simulink model "special_traj"  (R2018b)
settings: Solver=FixedStepDiscrete  StartTime=0.0  StopTime=10  FixedStep=Ts  RelTol=1e-3
InitFcn:
  | Ts = 0.001;
undefined symbols (not defined in the file or in its folder): DiscIntNeverNeededParam
libraries: powerlib_meascontrol x5, peGeneralControl x4
settings Model: Creator=Kamran  LastModifiedBy=Kamran
settings DebuggingCC: LibraryContextMissingDiagnostic=none
settings SFSimCC: SimUseLocalCustomCode=off
settings RTWCC: RTWUseLocalCustomCode=off

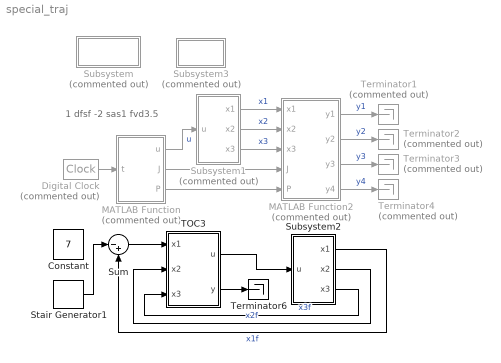
== system special_traj ==
  note: 1 dfsf -2 sas1 fvd3.5
  Constant : Constant  Value=7  SampleTime=Ts
  Digital Clock : DigitalClock  Commented=on  SampleTime=Ts
  MATLAB Function : MATLAB Function  Commented=on  TreatAsAtomicUnit=on
  MATLAB Function2 : MATLAB Function  Commented=on  TreatAsAtomicUnit=on
  Stair Generator1 : powerlib_meascontrol/Pulse & Signal Generators/Stair Generator  t=[0, 1, 5]  e=[1, 5, -3]  Ts=Ts
      settings: SourceProductName=Simscape Power Systems
  Subsystem : Subsystem  Commented=on
  Subsystem1 : Subsystem  Commented=on
  Subsystem2 : Subsystem  mask{X10=0, X20=0, X2M=inf, X30=0, X3M=1.5}
  Subsystem3 : Subsystem  Commented=on
  Sum : Sum  Inputs=|-+
  TOC3 : MATLAB Function  TreatAsAtomicUnit=on  SystemSampleTime=Ts
  Terminator{1..4} (4 alike) : Terminator  Commented=on
  Terminator6 : Terminator
  wires:
  MATLAB Function/1(u) -> Subsystem1/1(u)  "u"
  Digital Clock/1 -> MATLAB Function/1(t)
  MATLAB Function2/1(y1) -> Terminator1/1  "y1"
  Subsystem1/1(x1) -> MATLAB Function2/1(x1)  "x1"
  Subsystem1/2(x2) -> MATLAB Function2/2(x2)  "x2"
  Subsystem1/3(x3) -> MATLAB Function2/3(x3)  "x3"
  MATLAB Function2/2(y2) -> Terminator2/1  "y2"
  MATLAB Function/2(J) -> MATLAB Function2/4(J)
  MATLAB Function2/3(y3) -> Terminator3/1  "y3"
  MATLAB Function2/4(y4) -> Terminator4/1  "y4"
  MATLAB Function/3(P) -> MATLAB Function2/5(P)
  TOC3/1(u) -> Subsystem2/1(u)
  Subsystem2/1(x1) -> Sum/2  "x1f"
  Subsystem2/2(x2) -> TOC3/2(x2)  "x2f"
  Subsystem2/3(x3) -> TOC3/3(x3)  "x3f"
  TOC3/2(y) -> Terminator6/1
  Stair Generator1/1 -> Sum/1
  Sum/1 -> TOC3/1(x1)

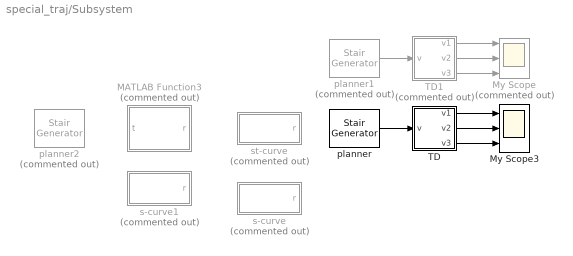
== system special_traj/Subsystem ==
  MATLAB Function3 : MATLAB Function  Commented=on  TreatAsAtomicUnit=on
  My Scope : Scope  Commented=on  NumInputPorts=3
  My Scope3 : Scope  NumInputPorts=3
  TD : Subsystem  mask{x3m=4, x2m=3}
      mask prompts: x3m "x3 max"; x2m "x2 max"
  TD1 : Subsystem  Commented=on  mask{J=1, A=1, D=0.5}
  planner : powerlib_meascontrol/Pulse & Signal Generators/Stair Generator  t=[0, 1, 4]  e=[0, 1, 0]  Ts=Ts
      settings: SourceProductName=Simscape Electrical
  planner1 : powerlib_meascontrol/Pulse & Signal Generators/Stair Generator  Commented=on  t=[0, 1, 5, 8]  e=[0, 1, 0.1, 0]  Ts=Ts
      settings: SourceProductName=Simscape Electrical
  planner2 : powerlib_meascontrol/Pulse & Signal Generators/Stair Generator  Commented=on  t=[0, 1.9, 6, 8.1]  e=[1, -1, 1, 0]  Ts=Ts
      settings: SourceProductName=Simscape Electrical
  s-curve : MATLAB Function  Commented=on  TreatAsAtomicUnit=on  mask{P=3, V=1, A=2, J=3, Ts=0.001}
  s-curve1 : MATLAB Function  Commented=on  TreatAsAtomicUnit=on  mask{P=0.5, V=1, A=1, D=2, J=3, I=6, Ts=0.001}
  st-curve : MATLAB Function  Commented=on  TreatAsAtomicUnit=on  mask{P=3, V=1, A=2, J=3, Ts=Ts}
  wires:
  TD/3(v3) -> My Scope3/3
  TD/2(v2) -> My Scope3/2
  TD1/2(v2) -> My Scope/2
  TD/1(v1) -> My Scope3/1
  planner1/1 -> TD1/1(v)
  TD1/3(v3) -> My Scope/3
  TD1/1(v1) -> My Scope/1
  planner/1 -> TD/1(v)

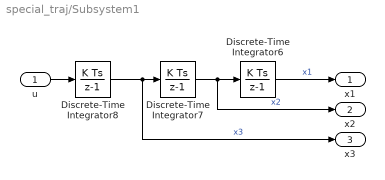
== system special_traj/Subsystem1 ==
  u : Inport
  Discrete-Time Integrator6 : DiscreteIntegrator  SampleTime=-1  ICPrevOutput=DiscIntNeverNeededParam  ICPrevScaledInput=DiscIntNeverNeededParam
  Discrete-Time Integrator7 : DiscreteIntegrator  SampleTime=-1  ICPrevOutput=DiscIntNeverNeededParam  ICPrevScaledInput=DiscIntNeverNeededParam
  Discrete-Time Integrator8 : DiscreteIntegrator  SampleTime=-1  ICPrevOutput=DiscIntNeverNeededParam  ICPrevScaledInput=DiscIntNeverNeededParam
  x1 : Outport
  x2 : Outport  Port=2
  x3 : Outport  Port=3
  wires:
  Discrete-Time Integrator8/1 -> x3/1, Discrete-Time Integrator7/1  "x3"
  Discrete-Time Integrator7/1 -> x2/1, Discrete-Time Integrator6/1  "x2"
  u/1 -> Discrete-Time Integrator8/1
  Discrete-Time Integrator6/1 -> x1/1  "x1"

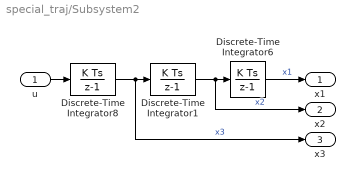
== system special_traj/Subsystem2 ==
  u : Inport
  Discrete-Time Integrator1 : DiscreteIntegrator  InitialCondition=X20  SampleTime=-1  LimitOutput=on  UpperSaturationLimit=X2M  LowerSaturationLimit=-X2M  ICPrevOutput=DiscIntNeverNeededParam  ICPrevScaledInput=DiscIntNeverNeededParam
  Discrete-Time Integrator6 : DiscreteIntegrator  InitialCondition=X10  SampleTime=-1  ICPrevOutput=DiscIntNeverNeededParam  ICPrevScaledInput=DiscIntNeverNeededParam
  Discrete-Time Integrator8 : DiscreteIntegrator  InitialCondition=X30  SampleTime=-1  LimitOutput=on  UpperSaturationLimit=X3M  LowerSaturationLimit=-X3M  ICPrevOutput=DiscIntNeverNeededParam  ICPrevScaledInput=DiscIntNeverNeededParam
  x1 : Outport
  x2 : Outport  Port=2
  x3 : Outport  Port=3
  wires:
  Discrete-Time Integrator8/1 -> x3/1, Discrete-Time Integrator1/1  "x3"
  Discrete-Time Integrator1/1 -> x2/1, Discrete-Time Integrator6/1  "x2"
  u/1 -> Discrete-Time Integrator8/1
  Discrete-Time Integrator6/1 -> x1/1  "x1"

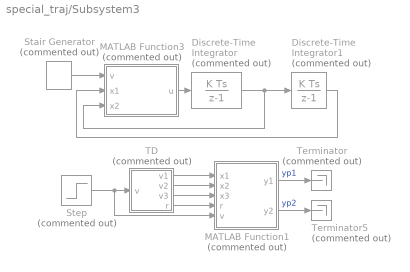
== system special_traj/Subsystem3 ==
  Discrete-Time Integrator : DiscreteIntegrator  Commented=on  SampleTime=-1  LimitOutput=on  UpperSaturationLimit=2  LowerSaturationLimit=-2  ICPrevOutput=DiscIntNeverNeededParam  ICPrevScaledInput=DiscIntNeverNeededParam
  Discrete-Time Integrator1 : DiscreteIntegrator  Commented=on  SampleTime=-1  ICPrevOutput=DiscIntNeverNeededParam  ICPrevScaledInput=DiscIntNeverNeededParam
  MATLAB Function1 : MATLAB Function  Commented=on  TreatAsAtomicUnit=on
  MATLAB Function3 : MATLAB Function  Commented=on  TreatAsAtomicUnit=on
  Stair Generator : powerlib_meascontrol/Pulse & Signal Generators/Stair Generator  Commented=on  t=[0, 1, 4]  e=[1, 5, -3]  Ts=Ts
      settings: SourceProductName=Simscape Power Systems
  Step : Step  Commented=on  After=3  SampleTime=Ts
  TD : Subsystem  Commented=on  mask{x3m=2, x2m=inf}
      mask prompts: x3m "x3 max"; x2m "x2 max"
  Terminator : Terminator  Commented=on
  Terminator5 : Terminator  Commented=on
  wires:
  Discrete-Time Integrator/1 -> MATLAB Function3/3(x2), Discrete-Time Integrator1/1
  Discrete-Time Integrator1/1 -> MATLAB Function3/2(x1)
  MATLAB Function3/1(u) -> Discrete-Time Integrator/1
  Stair Generator/1 -> MATLAB Function3/1(v)
  TD/4(r) -> MATLAB Function1/4(r)
  Step/1 -> MATLAB Function1/5(v), TD/1(v)
  TD/1(v1) -> MATLAB Function1/1(x1)
  MATLAB Function1/2(y2) -> Terminator5/1  "yp2"
  MATLAB Function1/1(y1) -> Terminator/1  "yp1"
  TD/2(v2) -> MATLAB Function1/2(x2)
  TD/3(v3) -> MATLAB Function1/3(x3)

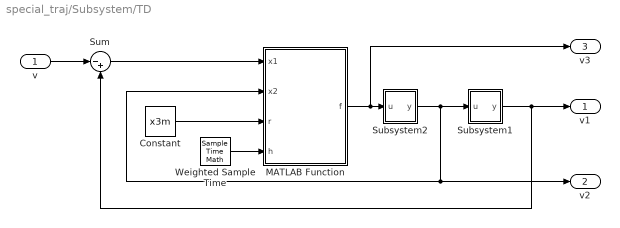
== system special_traj/Subsystem/TD ==
  v : Inport
  Constant : Constant  Value=x3m  SampleTime=-1
  MATLAB Function : MATLAB Function  TreatAsAtomicUnit=on
  Subsystem1 : Subsystem  mask{sat=inf, x0=0}
      mask Display: droots([], [0], 1);
  Subsystem2 : Subsystem  mask{sat=x2m, x0=0}
      mask Display: droots([], [0], 1);
  Sum : Sum  Inputs=|-+
  Weighted Sample Time : SampleTimeMath  TsampMathOp=Ts Only
  v1 : Outport
  v2 : Outport  Port=2
  v3 : Outport  Port=3
  wires:
  Subsystem2/1(y) -> Subsystem1/1(u), v2/1, MATLAB Function/2(x2)
  Subsystem1/1(y) -> Sum/2, v1/1
  v/1 -> Sum/1
  Weighted Sample Time/1 -> MATLAB Function/4(h)
  Sum/1 -> MATLAB Function/1(x1)
  Constant/1 -> MATLAB Function/3(r)
  MATLAB Function/1(f) -> v3/1, Subsystem2/1(u)

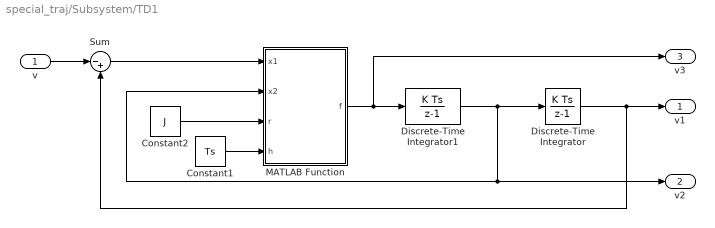
== system special_traj/Subsystem/TD1 ==
  v : Inport
  Constant1 : Constant  Value=Ts  SampleTime=-1
  Constant2 : Constant  Value=J  SampleTime=-1
  Discrete-Time Integrator : DiscreteIntegrator  SampleTime=-1  ICPrevOutput=DiscIntNeverNeededParam  ICPrevScaledInput=DiscIntNeverNeededParam
  Discrete-Time Integrator1 : DiscreteIntegrator  SampleTime=-1  LimitOutput=on  UpperSaturationLimit=A  LowerSaturationLimit=-D  ICPrevOutput=DiscIntNeverNeededParam  ICPrevScaledInput=DiscIntNeverNeededParam
  MATLAB Function : MATLAB Function  TreatAsAtomicUnit=on
  Sum : Sum  Inputs=|-+
  v1 : Outport
  v2 : Outport  Port=2
  v3 : Outport  Port=3
  wires:
  Discrete-Time Integrator/1 -> Sum/2, v1/1
  v/1 -> Sum/1
  Constant1/1 -> MATLAB Function/4(h)
  Sum/1 -> MATLAB Function/1(x1)
  MATLAB Function/1(f) -> v3/1, Discrete-Time Integrator1/1
  Discrete-Time Integrator1/1 -> Discrete-Time Integrator/1, v2/1, MATLAB Function/2(x2)
  Constant2/1 -> MATLAB Function/3(r)

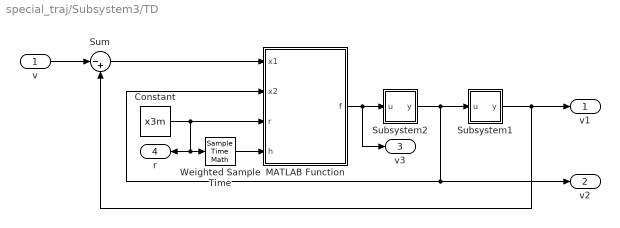
== system special_traj/Subsystem3/TD ==
  v : Inport
  Constant : Constant  Value=x3m  SampleTime=-1
  MATLAB Function : MATLAB Function  TreatAsAtomicUnit=on
  Subsystem1 : Subsystem  mask{sat=inf, x0=0}
      mask Display: droots([], [0], 1);
  Subsystem2 : Subsystem  mask{sat=x2m, x0=0}
      mask Display: droots([], [0], 1);
  Sum : Sum  Inputs=|-+
  Weighted Sample Time : SampleTimeMath  TsampMathOp=Ts Only
  v1 : Outport
  v2 : Outport  Port=2
  v3 : Outport  Port=3
  r : Outport  Port=4
  wires:
  Subsystem2/1(y) -> Subsystem1/1(u), v2/1, MATLAB Function/2(x2)
  Subsystem1/1(y) -> Sum/2, v1/1
  v/1 -> Sum/1
  Weighted Sample Time/1 -> MATLAB Function/4(h)
  Sum/1 -> MATLAB Function/1(x1)
  MATLAB Function/1(f) -> v3/1, Subsystem2/1(u)
  Constant/1 -> r/1, Weighted Sample Time/1, MATLAB Function/3(r)

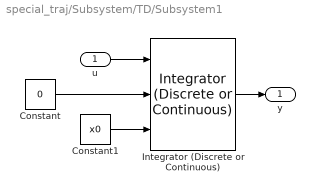
== system special_traj/Subsystem/TD/Subsystem1 ==
  u : Inport
  Constant : Constant  Value=0
  Constant1 : Constant  Value=x0
  Integrator (Discrete or Continuous) : peGeneralControl/Integrator (Discrete or Continuous)  LabelModeActiveChoice=Discrete  ExternalReset=level  LimitType=Anti-windup  B=sat  A=-sat  Ts=-1
  y : Outport
  wires:
  Constant1/1 -> Integrator (Discrete or Continuous)/3
  u/1 -> Integrator (Discrete or Continuous)/1
  Constant/1 -> Integrator (Discrete or Continuous)/2
  Integrator (Discrete or Continuous)/1 -> y/1

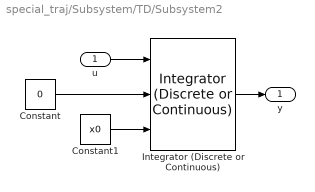
== system special_traj/Subsystem/TD/Subsystem2 ==
  u : Inport
  Constant : Constant  Value=0
  Constant1 : Constant  Value=x0
  Integrator (Discrete or Continuous) : peGeneralControl/Integrator (Discrete or Continuous)  LabelModeActiveChoice=Discrete  ExternalReset=level  LimitType=Anti-windup  B=sat  A=-sat  Ts=-1
  y : Outport
  wires:
  Integrator (Discrete or Continuous)/1 -> y/1
  Constant/1 -> Integrator (Discrete or Continuous)/2
  u/1 -> Integrator (Discrete or Continuous)/1
  Constant1/1 -> Integrator (Discrete or Continuous)/3

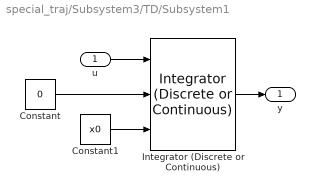
== system special_traj/Subsystem3/TD/Subsystem1 ==
  u : Inport
  Constant : Constant  Value=0
  Constant1 : Constant  Value=x0
  Integrator (Discrete or Continuous) : peGeneralControl/Integrator (Discrete or Continuous)  LabelModeActiveChoice=Discrete  ExternalReset=level  LimitType=Anti-windup  B=sat  A=-sat  Ts=-1
  y : Outport
  wires:
  Constant1/1 -> Integrator (Discrete or Continuous)/3
  u/1 -> Integrator (Discrete or Continuous)/1
  Constant/1 -> Integrator (Discrete or Continuous)/2
  Integrator (Discrete or Continuous)/1 -> y/1

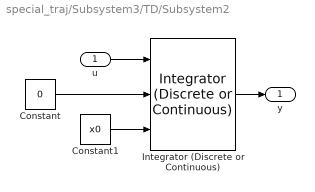
== system special_traj/Subsystem3/TD/Subsystem2 ==
  u : Inport
  Constant : Constant  Value=0
  Constant1 : Constant  Value=x0
  Integrator (Discrete or Continuous) : peGeneralControl/Integrator (Discrete or Continuous)  LabelModeActiveChoice=Discrete  ExternalReset=level  LimitType=Anti-windup  B=sat  A=-sat  Ts=-1
  y : Outport
  wires:
  Integrator (Discrete or Continuous)/1 -> y/1
  Constant/1 -> Integrator (Discrete or Continuous)/2
  u/1 -> Integrator (Discrete or Continuous)/1
  Constant1/1 -> Integrator (Discrete or Continuous)/3

== matlab function special_traj/Subsystem/s-curve1 ==
  data: r output; P parameter; V parameter; A parameter; D parameter; J parameter; I parameter; Ts parameter
function r = profile(P, V, A, D, J, I, Ts)

persistent t;
if isempty(t)
    t = 0;
else
    t = t + Ts;
end

if P/V < (A/J/2 + V/A/2 + D/I/2 + V/D/2)
    a = 1/A + 1/D;
    b = A/J + D/I;
    c = -2*P;
    V = -b + sqrt(b^2 - 4*a*c)/2/a;
end

if V*J < A^2
    A = sqrt(V*J);
end

if V*I < D^2
    D = sqrt(V*I);
end

t1 = A/J;
t2 = V/A - A/J;
t3 = P/V - A/J/2 - V/A/2 - D/I/2 - V/D/2;
t4 = D/I;
t5 = V/D - D/I;

% t1 = A/J;
% t4 = D/I;
% t2 = V/A - t1;
% t5 = V/D - t4;
% t3 = P/V - t2/2 - t1 - t5/2 - t4;

% t  = round(t  / Ts) * Ts;
t1 = round(t1 / Ts) * Ts;
t2 = round(t2 / Ts) * Ts;
t3 = round(t3 / Ts) * Ts;
t4 = round(t4 / Ts) * Ts;
t5 = round(t5 / Ts) * Ts;

% K = 2*P/(t1*(t1+t2)*(t5+2*t4+2*t3+2*t1+t2));

if 0
elseif t < (t1)
    r = +J;
elseif t < (t1 + t2)
    r = 0;
elseif t < (2*t1 + t2)
    r = -J;
elseif t < (2*t1 + t2 + t3)
    r = 0;
elseif t < (2*t1 + t2 + t3 + t4)
    r = -I;
elseif t < (2*t1 + t2 + t3 + t4 + t5)
    r = 0;
elseif t < (2*t1 + t2 + t3 + 2*t4 + t5)
    r = I;
else
    r = 0;
end

end

== matlab function special_traj/Subsystem/TD1/MATLAB Function ==
  data: x1 input; f output; x2 input; r input; h input
function f = fhan(x1, x2, r, h)

    d = r * h^2;
    a0 = h * x2;
    y = x1 + a0;
    a1 = sqrt(d * (d + 8 * abs(y)));
    a2 = a0 + sign(y) * (a1 - d) / 2;
    sy = (sign(y + d) - sign(y - d)) / 2;
    a = (a0 + y - a2) * sy + a2;
    sa = (sign(a + d) - sign(a - d)) / 2;
    f = -r * (a / d - sign(a)) * sa - r * sign(a);

end

== matlab function special_traj/Subsystem/s-curve ==
  data: r output; P parameter; V parameter; A parameter; J parameter; Ts parameter
function r = profile(P, V, A, J, Ts)

persistent t;
if isempty(t)
    t = 0;
else
    t = t + Ts;
end

if P/V < (A/J + V/A)
    b = A/J;
    V = A * (-b + sqrt(b^2 + 4*P/A)) / 2;
end

if V*J < A^2
    A = sqrt(J*V);
end

t1 = A/J;
t2 = V/A - A/J;
t3 = P/V - V/A - A/J;
t4 = t1;
t5 = t2;

t = round(t / Ts) * Ts;
t1 = round(t1 / Ts) * Ts;
t2 = round(t2 / Ts) * Ts;
t3 = round(t3 / Ts) * Ts;
t4 = round(t4 / Ts) * Ts;
t5 = round(t5 / Ts) * Ts;

K = 2*P/(t1*(t1+t2)*(t5+2*t4+2*t3+2*t1+t2));

if 0
elseif t < (t1)
    r = +K;
elseif t < (t1 + t2)
    r = 0;
elseif t < (2*t1 + t2)
    r = -K;
elseif t < (2*t1 + t2 + t3)
    r = 0;
elseif t < (2*t1 + t2 + t3 + t4)
    r = -K;
elseif t < (2*t1 + t2 + t3 + t4 + t5)
    r = 0;
elseif t < (2*t1 + t2 + t3 + 2*t4 + t5)
    r = K;
else
    r = 0;
end

end

== matlab function special_traj/Subsystem/TD/MATLAB Function ==
  data: x1 input; f output; x2 input; r input; h input
function f = fhan(x1, x2, r, h)

    d = r * h^2;
    a0 = h * x2;
    y = x1 + a0;
    a1 = sqrt(d * (d + 8 * abs(y)));
    a2 = a0 + sign(y) * (a1 - d) / 2;
    sy = (sign(y + d) - sign(y - d)) / 2;
    a = (a0 + y - a2) * sy + a2;
    sa = (sign(a + d) - sign(a - d)) / 2;
    f = -r * (a / d - sign(a)) * sa - r * sign(a);

end

== matlab function special_traj/Subsystem/MATLAB Function3 ==
  data: t input; r output
function r = fcn(t)

P = 15;
J = 1;
I = J;
A = 1;
D = A;
V = 1;

t1 = A/J;
t2 = V/A - A/J;
t3 = P/V - A/J/2 - V/A/2 - D/I/2 - V/D/2;
t4 = D/I;
t5 = V/D - D/I;

ro = D/A;
con1 = V >= (A^2/J);
con2 = V >= (D^2/I);
con3 = P/V >= (D/2/J/ro + ro*V/2/D + D/2/J + V/2/D);
con4 = P/V >= ((1+1/ro)*D/2/J + (ro+1)*V/2/D);

if ~con1 || ~con2 || ~con3 || ~con4
    r = 0;
elseif t < (t1)
    r = +1;
elseif t < (t1 + t2)
    r = 0;
elseif t < (2*t1 + t2)
    r = -1;
elseif t < (2*t1 + t2 + t3)
    r = 0;
elseif t < (2*t1 + t2 + t3 + t4)
    r = -1;
elseif t < (2*t1 + t2 + t3 + t4 + t5)
    r = 0;
elseif t < (2*t1 + t2 + t3 + 2*t4 + t5)
    r = 1;
else
    r = 0;
end

end

== matlab function special_traj/Subsystem/st-curve ==
  data: r output; P parameter; V parameter; A parameter; J parameter; Ts parameter
function r = profile(P, V, A, J, Ts)

persistent t;
if isempty(t)
    t = 0;
else
    t = t + Ts;
end

if P/V < 3*A/2/J + V/A
    b = 3*A/2/J;
    V = A * (-b + sqrt(b^2 + 4*P/A)) / 2;
end

if 2*J*V < 3*A^2
    A = sqrt(2*J*V/3);
end

t1 = 3*A/2/J;
t2 = V/A - t1;
t3 = P/V - V/A - t1;
t4 = t1;
t5 = t2;

t = round(t / Ts) * Ts;
t1 = round(t1 / Ts) * Ts;
t2 = round(t2 / Ts) * Ts;
t3 = round(t3 / Ts) * Ts;
t4 = round(t4 / Ts) * Ts;
t5 = round(t5 / Ts) * Ts;

K = 12*P/(t1^3*(t1+t2)*(t5+2*t4+2*t3+2*t1+t2));

if 0
elseif t < (t1)
    tt = t;
    ss = tt*(t1-tt);
    r = +K*ss;
elseif t < (t1 + t2)
    r = 0;
elseif t < (2*t1 + t2)
    tt = t - (t1 + t2);
    ss = tt*(t1-tt);
    r = -K*ss;
elseif t < (2*t1 + t2 + t3)
    r = 0;
elseif t < (2*t1 + t2 + t3 + t4)
    tt = t - (2*t1 + t2 + t3);
    ss = tt*(t1-tt);
    r = -K*ss;
elseif t < (2*t1 + t2 + t3 + t4 + t5)
    r = 0;
elseif t < (2*t1 + t2 + t3 + 2*t4 + t5)
    tt = t - (2*t1 + t2 + t3 + t4 + t5);
    ss = tt*(t1-tt);
    r = K*ss;
else
    r = 0;
end

end

== matlab function special_traj/MATLAB Function ==
  data: t input; u output; J output; P output
function [u, J, P] = fcn(t)

S = 1;
P = 6*S;
J = 4*S;
O = 0;
T = nthroot(P/J/2,3);

t = t - O;

if (t<0)
    u = 0;
elseif (t<T)
    u = +J;
elseif (t<3*T)
    u = -J;
elseif (t<4*T)
    u = +J;
else
    u = 0;
end

== matlab function special_traj/Subsystem3/TD/MATLAB Function ==
  data: x1 input; f output; x2 input; r input; h input
function f = fhan(x1, x2, r, h)

    d = r * h^2;
    a0 = h * x2;
    y = x1 + a0;
    a1 = sqrt(d * (d + 8 * abs(y)));
    a2 = a0 + sign(y) * (a1 - d) / 2;
    sy = (sign(y + d) - sign(y - d)) / 2;
    a = (a0 + y - a2) * sy + a2;
    sa = (sign(a + d) - sign(a - d)) / 2;
    f = -r * (a / d - sign(a)) * sa - r * sign(a);
    
%     f = -sign(x1 + .5*x2*abs(x2));

end

== matlab function special_traj/Subsystem3/MATLAB Function1 ==
  data: x1 input; x2 input; x3 input; r input; y1 output; v input; y2 output
function [y1, y2] = fcn(x1, x2, x3, r, v)
%   y = -sat(x1 - v + x2*abs(x2)/2);
    e = v - x1;
    
    y1 = -e + x2*abs(x2)/2/r;
    y2 = -e - x2*abs(x2)/2/r;
    
%     y1 = -e + x2^2/2;
%     y2 = -e - x2^2/2;
end

function y = sat(s)
    psi = eps;
    if (abs(s) > psi)
        y = sign(s);
    else
        y = s / psi;
    end
end

== matlab function special_traj/MATLAB Function2 ==
  data: x1 input; x2 input; x3 input; J input; y1 output; y2 output; y3 output; y4 output; P input
function [y1, y2, y3, y4] = fcn(x1, x2, x3, J, P)
    r = abs(J);
    e = P - x1;
    
    y1 = -e + x3^3/3/r^2 + x3*abs(x2)/r;
    y2 = -e + x3^3/3/r^2 - x3*abs(x2)/r;
    
    y3 = x2 + x3*abs(x3)/2/r;
    y4 = x2 - x3*abs(x3)/2/r;
    
    y3 = sign(x2) * (abs(x2) + x3^2/2/r);
    y4 = sign(x2) * (abs(x2) - x3^2/2/r);
    
    xc = y1 + y3*sqrt(abs(y3)/r);
    
%     y1 = -e + x3^3/3/r^2 + x2*x3/r;
%     y2 = -e + x3^3/3/r^2 - x2*x3/r;
%     y3 = x2 + x3^2/2/r;
%     y4 = x2 - x3^2/2/r;
end

== matlab function special_traj/TOC3 ==
  data: u output; x1 input; x2 input; x3 input; y output
function [u, y] = fcn(x1, x2, x3)
    r = 2.5;
    h = 0.001;
    vm = 2.5;
    
    y1 = x1  + x3^3/3/r^2 + x3*abs(x2)/r;
    y3 = sign(x2) * (abs(x2) + x3^2/2/r);
    pcan = y3*sqrt(abs(y3)/r);
    xcal = y1 + pcan;
    y4 = x2 + x3*abs(x3)/2/r;
    y = [xcal y4];
    
%     u = fhan(x2, x3, r, h);
    
    if abs(y3) > vm && sign(x2) == sign(x3)
        u = -r*sign(y3);
    elseif abs(xcal) > 0.5
        u = -r * sign(xcal);
    else
        u = fhan(x2, x3, r, h);
%         u = -r * sign(y4);
    end

%     b1 = xcalc(-e+x2*h*2, x2+x3*h*2, x3+r*h*2, 0.9*r);% estimate(-e, x2, x3, -r, r*1.1, h);
%     b2 = xcalc(-e+x2*h*2, x2+x3*h*2, x3+r*h*2, 1.1*r);% estimate(-e, x2, x3, -r, r*0.9, h);
%     kk=r;
%    if(sign(b1)~=sign(b2))
%         kk =  (1-0.1*(b1 + b2) / (b1 - b2))*r;
%    end
%    
%     a1 = estimate(-e, x2, x3, +kk, kk, h);
%     a2 = estimate(-e, x2, x3, -kk, kk, h);
%     a0 = estimate(-e, x2, x3,  0, kk, h);
% 
%     y = [a1 a2 a0 b1 b2 kk];
% 
%         u = -kk * (a1 + a2) / (a1 - a2);
%         if abs(u) > kk
%             u = kk * sign(u);
%         end

    %if(sign(a1)==sign(a2))
    %    u= -r*sign(abs(a1)-abs(a2))*1.02;
    %else
            %u=-(abs(a1)*r+abs(a2)*-r)/(abs(a1)+abs(a2));
    %end
    
%     if abs(y3) > vm && sign(y3) == sign(x3)
%         u = -r*sign(y3);
%     elseif abs(xcal) > 0.05
%         u = -r * sign(xcal);
%     else
%         u = fhan(x2, x3, r, h);
% %         u = -r * sign(y4);
%     end
end

function xc = estimate1(x1, x2, x3, rs, jmax, h)
    d1 = x1 + x2 * h;
    d2 = x2 + x3 * h;
    d3 = x3 + rs * h;
    xc = xcalc(d1, d2, d3, jmax);
end

function xc = estimate2(x1, x2, x3, rs, jmax, h)
    d1 = x1 + x2 * h;
    d2 = x2 + x3 * h;
    d3 = x3 + rs * h;
    d1 = d1 + d2 * h;
    d2 = d2 + d3 * h;
    d3 = d3 - rs * h;
    xc = xcalc(d1, d2, d3, jmax);
end

function xc = xcalc(x1, x2, x3, r)
    y1 = x1 + x3^3/3/r^2 + x3*abs(x2)/r;
    y3 = sign(x2) * (abs(x2) + x3^2/2/r);
    xc = y1 + y3*sqrt(abs(y3)/r);
end

function f = fhan(x1, x2, r, h)
    d = r * h^2;
    a0 = h * x2;
    y = x1 + a0;
    a1 = sqrt(d * (d + 8 * abs(y)));
    a2 = a0 + sign(y) * (a1 - d) / 2;
    sy = (sign(y + d) - sign(y - d)) / 2;
    a = (a0 + y - a2) * sy + a2;
    sa = (sign(a + d) - sign(a - d)) / 2;
    f = -r * (a / d - sign(a)) * sa - r * sign(a);
end

%     syms J;
%     x3x = x3 + J * h;
%     x2x = x2 + x3 * h + J*h^2 /2;
%     x1x = x1 + x2 * h + x3 *h^2/2 + J*h^3/6;
%     vm = x2x + x3^2/2*u;
%     xc = x3x^3/3/J^2 + x2x*x3x/J + vm*sart(abs(vm)/J);
% solve (J)...
%     A =

== matlab function special_traj/Subsystem3/MATLAB Function3 ==
  data: v input; u output; x1 input; x2 input
function u = fcn(v, x1, x2)
    r = 3;
    h = eps;
    e = v - x1;
    y1 = -e + x2*abs(x2)/2/r;
    y2 = -e - x2*abs(x2)/2/r;
    
    if abs(y1) > h
        u = -r * sign(y1); %%%%%%%%%%%%%%%%%%%%%%%%%%%%%%%
    else
        if abs(y2) > h
            u = -r * sign(y2);
        else
            u = 0;
        end
    end
end
